simulink model "modele_cheville_eleve"  (R2016a)
settings: Solver=ode45  StartTime=0.0  StopTime=1  RelTol=1e-3
PreLoadFcn:
  | ki=1;
  | ke=1;
  | L=2;
  | R=1;
  | kred=5;
  | Jeq=1;
  | f=1;
StartFcn:
  | ki=19.4e-3;
  | ke=19.4e-3;
  | L=0.6e-3;
  | R=5.4;
  | kred=130;
  | Jeq=0.015;
  | f=0;
settings Model: Creator=pt_ptsi  LastModifiedBy=pt_ptsi
settings DataIOCC: LimitDataPoints=on  SaveFormat=Array
settings DebuggingCC: UnderspecifiedInitializationDetection=Classic  MergeDetectMultiDrivingBlocksExec=none  SolverPrmCheckMsg=warning  AllowSymbolicDim=off  StateNameClashWarn=warning
settings HardwareCC: ProdBitPerPointer=32  ProdLargestAtomicFloat=None  ProdIntDivRoundTo=Undefined  ProdEndianess=Unspecified  ProdWordSize=32  ProdHWDeviceType=32-bit Generic
settings ModelReferenceCC: PropagateSignalLabelsOutOfModel=off
settings ConfigComp: CovModelRefEnable=Off

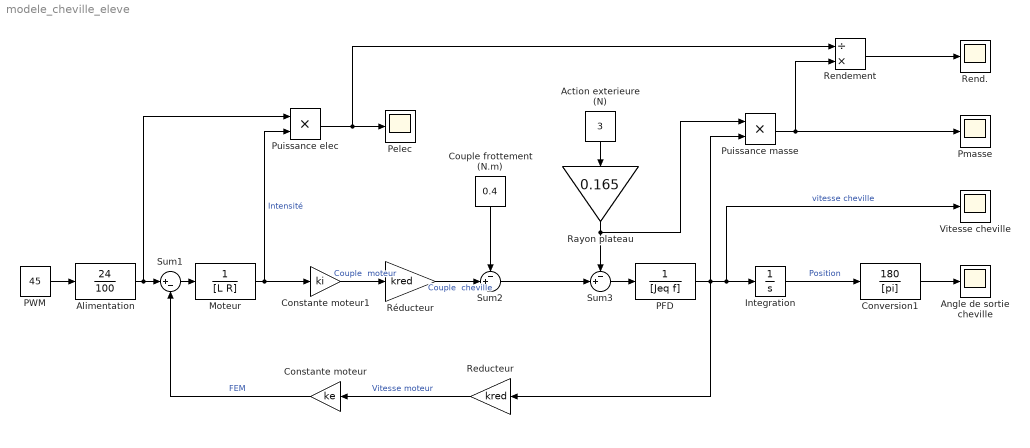
== system modele_cheville_eleve ==
  Action exterieure (N) : Constant  Value=3
  Alimentation : TransferFcn  Numerator=[24]  Denominator=[100]
  Angle de sortie cheville : Scope
  Constante moteur : Gain  Gain=ke
  Constante moteur1 : Gain  Gain=ki
  Conversion1 : TransferFcn  Numerator=[180]  Denominator=[pi]
  Couple frottement (N.m) : Constant  Value=0.4
  Integration : Integrator
  Moteur : TransferFcn  Denominator=[L R]
  PFD : TransferFcn  Denominator=[Jeq f]
  PWM : Constant  Value=45
  Pelec : Scope
  Pmasse : Scope
  Puissance elec : Product
  Puissance masse : Product
  Rayon plateau : Gain  Gain=0.165
  Reducteur : Gain  Gain=kred
  Rend. : Scope
  Rendement : Product  Inputs=/*
  Réducteur : Gain  Gain=kred
  Sum1 : Sum  Inputs=|+-
  Sum2 : Sum  Inputs=-+|
  Sum3 : Sum  Inputs=-+|
  Vitesse cheville : Scope
  wires:
  PWM/1 -> Alimentation/1
  Sum1/1 -> Moteur/1
  Moteur/1 -> Puissance elec/2, Constante moteur1/1  "Intensité"
  Réducteur/1 -> Sum2/2  "Couple  cheville"
  Sum2/1 -> Sum3/2
  Sum3/1 -> PFD/1
  Couple frottement (N.m)/1 -> Sum2/1
  Action exterieure (N)/1 -> Rayon plateau/1
  Constante moteur/1 -> Sum1/2  "FEM"
  Reducteur/1 -> Constante moteur/1  "Vitesse moteur"
  PFD/1 -> Puissance masse/2, Vitesse cheville/1, Integration/1, Reducteur/1  "vitesse cheville"
  Integration/1 -> Conversion1/1  "Position"
  Alimentation/1 -> Puissance elec/1, Sum1/1
  Conversion1/1 -> Angle de sortie cheville/1
  Rayon plateau/1 -> Puissance masse/1, Sum3/1
  Constante moteur1/1 -> Réducteur/1  "Couple  moteur"
  Puissance elec/1 -> Rendement/1, Pelec/1
  Puissance masse/1 -> Rendement/2, Pmasse/1
  Rendement/1 -> Rend./1
